simulink model "counter"  (R2023a)
settings: Solver=VariableStepAuto  StartTime=0.0  StopTime=30  RelTol=1e-3
libraries: simulink_extras x14
settings Model: Creator=prath  LastModifiedBy=prath

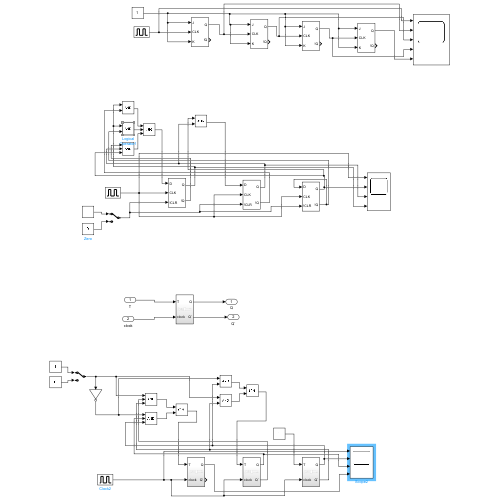
[thumbnail: Simulink's stored preview of the top-level diagram]
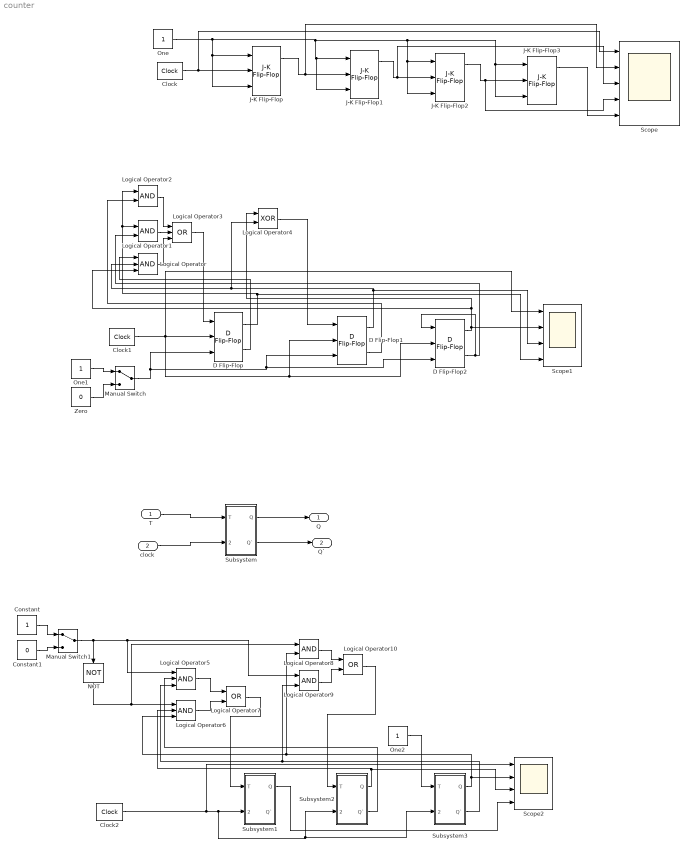
== system counter ==
  T : Inport
  clock : Inport  Port=2
  Clock : simulink_extras/Flip Flops/Clock  period=2
  Clock1 : simulink_extras/Flip Flops/Clock  period=2
  Clock2 : simulink_extras/Flip Flops/Clock  period=2
  Constant : Constant
  Constant1 : Constant  Value=0
  D Flip-Flop : simulink_extras/Flip Flops/D Flip-Flop
  D Flip-Flop1 : simulink_extras/Flip Flops/D Flip-Flop
  D Flip-Flop2 : simulink_extras/Flip Flops/D Flip-Flop
  J-K Flip-Flop{,1..3} (4 alike) : simulink_extras/Flip Flops/J-K Flip-Flop  initial_condition=0
  Logical Operator : Logic  Inputs=3  AllPortsSameDT=off  OutDataTypeStr=boolean
  Logical Operator{1..2,8..9} (4 alike) : Logic  AllPortsSameDT=off  OutDataTypeStr=boolean
  Logical Operator10 : Logic  Operator=OR  AllPortsSameDT=off  OutDataTypeStr=boolean
  Logical Operator3 : Logic  Operator=OR  Inputs=3  AllPortsSameDT=off  OutDataTypeStr=boolean
  Logical Operator4 : Logic  Operator=XOR  AllPortsSameDT=off  OutDataTypeStr=boolean
  Logical Operator5 : Logic  Inputs=3  AllPortsSameDT=off  OutDataTypeStr=boolean
  Logical Operator6 : Logic  Inputs=3  AllPortsSameDT=off  OutDataTypeStr=boolean
  Logical Operator7 : Logic  Operator=OR  AllPortsSameDT=off  OutDataTypeStr=boolean
  Manual Switch : ManualSwitch
  Manual Switch1 : ManualSwitch
  NOT : Logic  Operator=NOT  IconShape=distinctive  AllPortsSameDT=off  OutDataTypeStr=boolean
  One : Constant  OutDataTypeStr=Inherit: Inherit via back propagation
  One1 : Constant  OutDataTypeStr=Inherit: Inherit via back propagation
  One2 : Constant  OutDataTypeStr=Inherit: Inherit via back propagation
  Scope : Scope  NumInputPorts=5
  Scope1 : Scope  NumInputPorts=4
  Scope2 : Scope  NumInputPorts=4
  Subsystem : Subsystem
  Subsystem1 : Subsystem
  Subsystem2 : Subsystem
  Subsystem3 : Subsystem
  Zero : Constant  Value=0  OutDataTypeStr=Inherit: Inherit via back propagation
  Q : Outport
  Q` : Outport  Port=2
  wires:
  Clock/1 -> Scope/1, J-K Flip-Flop/2
  One/1 -> J-K Flip-Flop3/3, J-K Flip-Flop3/1, J-K Flip-Flop2/3, J-K Flip-Flop2/1, J-K Flip-Flop1/3, J-K Flip-Flop1/1, J-K Flip-Flop/3, J-K Flip-Flop/1
  J-K Flip-Flop/1 -> Scope/2, J-K Flip-Flop1/2
  J-K Flip-Flop1/1 -> Scope/3, J-K Flip-Flop2/2
  J-K Flip-Flop2/1 -> Scope/4, J-K Flip-Flop3/2
  J-K Flip-Flop3/1 -> Scope/5
  Clock1/1 -> Scope1/1, D Flip-Flop2/2, D Flip-Flop1/2, D Flip-Flop/2
  D Flip-Flop/1 -> Scope1/4, Logical Operator1/1, Logical Operator2/1
  D Flip-Flop1/2 -> Logical Operator2/2
  D Flip-Flop2/2 -> D Flip-Flop2/1, Logical Operator1/2
  D Flip-Flop/2 -> Logical Operator/1
  D Flip-Flop1/1 -> Scope1/3, Logical Operator4/2, Logical Operator/2
  D Flip-Flop2/1 -> Scope1/2, Logical Operator4/1, Logical Operator/3
  Logical Operator2/1 -> Logical Operator3/1
  Logical Operator1/1 -> Logical Operator3/2
  Logical Operator/1 -> Logical Operator3/3
  Logical Operator3/1 -> D Flip-Flop/1
  Logical Operator4/1 -> D Flip-Flop1/1
  One1/1 -> Manual Switch/1
  Zero/1 -> Manual Switch/2
  Manual Switch/1 -> D Flip-Flop2/3, D Flip-Flop1/3, D Flip-Flop/3
  T/1 -> Subsystem/1(T)
  clock/1 -> Subsystem/2(clock)
  Subsystem/1(Q) -> Q/1
  Subsystem/2(Q`) -> Q`/1
  One2/1 -> Subsystem3/1(T)
  Constant/1 -> Manual Switch1/1
  Constant1/1 -> Manual Switch1/2
  Manual Switch1/1 -> NOT/1, Logical Operator9/1, Logical Operator5/1
  Subsystem2/2(Q`) -> Logical Operator5/2
  Subsystem3/2(Q`) -> Logical Operator9/2, Logical Operator5/3
  NOT/1 -> Logical Operator8/1, Logical Operator6/1
  Subsystem2/1(Q) -> Scope2/3, Logical Operator6/2
  Subsystem3/1(Q) -> Scope2/2, Logical Operator8/2, Logical Operator6/3
  Logical Operator6/1 -> Logical Operator7/2
  Logical Operator5/1 -> Logical Operator7/1
  Logical Operator7/1 -> Subsystem1/1(T)
  Clock2/1 -> Scope2/1, Subsystem3/2(clock), Subsystem2/2(clock), Subsystem1/2(clock)
  Subsystem1/1(Q) -> Scope2/4
  Logical Operator8/1 -> Logical Operator10/1
  Logical Operator9/1 -> Logical Operator10/2
  Logical Operator10/1 -> Subsystem2/1(T)

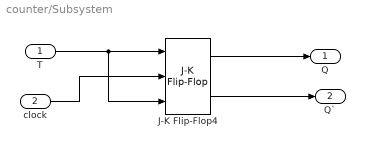
== system counter/Subsystem ==
  T : Inport
  clock : Inport  Port=2
  J-K Flip-Flop4 : simulink_extras/Flip Flops/J-K Flip-Flop  initial_condition=0
  Q : Outport
  Q` : Outport  Port=2
  wires:
  clock/1 -> J-K Flip-Flop4/2
  J-K Flip-Flop4/1 -> Q/1
  J-K Flip-Flop4/2 -> Q`/1
  T/1 -> J-K Flip-Flop4/3, J-K Flip-Flop4/1

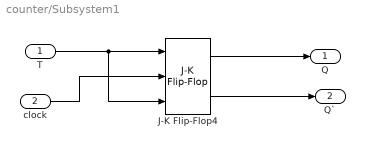
== system counter/Subsystem1 ==
  T : Inport
  clock : Inport  Port=2
  J-K Flip-Flop4 : simulink_extras/Flip Flops/J-K Flip-Flop  initial_condition=0
  Q : Outport
  Q` : Outport  Port=2
  wires:
  clock/1 -> J-K Flip-Flop4/2
  J-K Flip-Flop4/1 -> Q/1
  J-K Flip-Flop4/2 -> Q`/1
  T/1 -> J-K Flip-Flop4/3, J-K Flip-Flop4/1

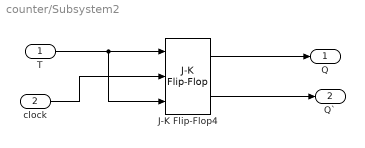
== system counter/Subsystem2 ==
  T : Inport
  clock : Inport  Port=2
  J-K Flip-Flop4 : simulink_extras/Flip Flops/J-K Flip-Flop  initial_condition=0
  Q : Outport
  Q` : Outport  Port=2
  wires:
  clock/1 -> J-K Flip-Flop4/2
  J-K Flip-Flop4/1 -> Q/1
  J-K Flip-Flop4/2 -> Q`/1
  T/1 -> J-K Flip-Flop4/3, J-K Flip-Flop4/1

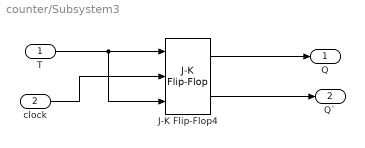
== system counter/Subsystem3 ==
  T : Inport
  clock : Inport  Port=2
  J-K Flip-Flop4 : simulink_extras/Flip Flops/J-K Flip-Flop  initial_condition=0
  Q : Outport
  Q` : Outport  Port=2
  wires:
  clock/1 -> J-K Flip-Flop4/2
  J-K Flip-Flop4/1 -> Q/1
  J-K Flip-Flop4/2 -> Q`/1
  T/1 -> J-K Flip-Flop4/3, J-K Flip-Flop4/1
